simulink model "inverse_kinematics"  (R2021b)
settings: Solver=ode1  StartTime=0.0  StopTime=inf  FixedStep=0.01  RelTol=1e-3
undefined symbols (not defined in the file): Levenberg, Marquardt, W, X, Y, Z
libraries: robotlib x6, simulink x2, robotcorelib x1, robotmaniplib x1
settings Model: Creator=alessandrini  LastModifiedBy=alessandrini
settings SolverCC: AlgebraicLoopSolver=TrustRegion
settings OptimizationCC: EnhancedBackFolding=on  PassReuseOutputArgsThreshold=0  MaxStackSize=64  OptimizeBlockOrder=speed  DifferentSizesBufferReuse=on  OptimizationCustomize=off
settings DebuggingCC: ParameterTunabilityLossMsg=error  SFMachineParentedDataDiag=warning
settings HardwareCC: ProdBitPerPointer=32  ProdBitPerSizeT=32  ProdBitPerPtrDiffT=32  ProdLargestAtomicFloat=None  ProdIntDivRoundTo=Undefined  ProdEndianess=Unspecified  ProdWordSize=32  ProdHWDeviceType=Generic->Unspecified (assume 32-bit Generic)  UseEmbeddedCoderFeatures=off
settings RTWCC: Description=Embedded Coder  SystemTargetFile=ert.tlc  HardwareBoard=Robot Operating System (ROS)  TLCOptions="-aInlineSetEventsForThisBaseRateFcn=TLC_FALSE -aSuppressMultiTaskScheduler=TLC_FALSE  -aRateBasedStepFcn=0"  TemplateMakefile=ert_default_tmf  Toolchain=Catkin  TargetLang=C++
settings CodeAppCC: ForceParamTrailComments=on  OperatorAnnotations=on
settings ERTTargetCC: ERTCustomFileBanners=off  SupportContinuousTime=on  SupportNonInlinedSFcns=on  RemoveResetFunc=off  ModelStepFunctionPrototypeControlCompliant=off

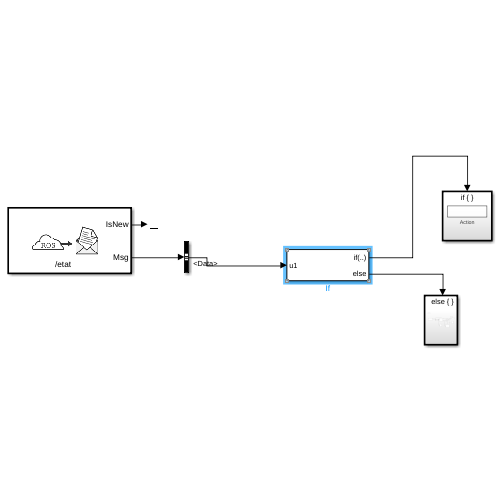
[thumbnail: Simulink's stored preview of the top-level diagram]
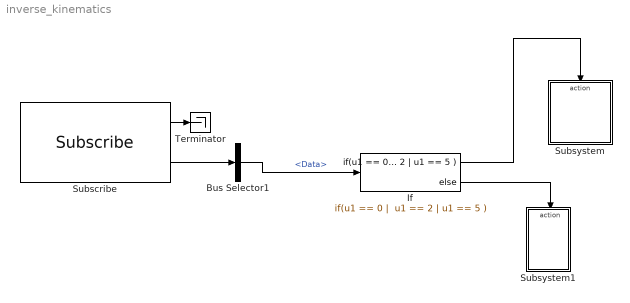
== system inverse_kinematics ==
  Bus Selector1 : BusSelector  OutputSignals=Data
  If : If  IfExpression="u1 == 0 |  u1 == 2 | u1 == 5"
  Subscribe : robotlib/Subscribe  topicSource=Specify your own  topic=/etat  messageType=std_msgs/Int16  SampleTime=-1  legacyBusStruct=off  messageQueueLength=1
  Subsystem : Subsystem
  Subsystem1 : Subsystem
  Terminator : Terminator
  wires:
  Subscribe/2 -> Bus Selector1/1
  Subscribe/1 -> Terminator/1
  Bus Selector1/1 -> If/1  "<Data>"
  If/1 -> Subsystem/Action
  If/2 -> Subsystem1/Action

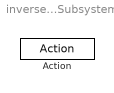
== system inverse_kinematics/Subsystem ==
  Action : ActionPort  InitializeStates=reset  ActionPortLabel="if(u1 == 0 |  u1 == 2 | u1 == 5 )"

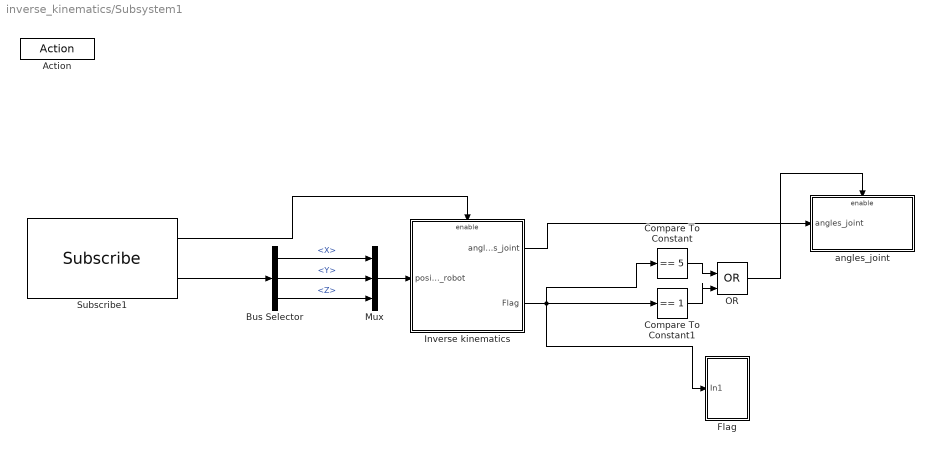
== system inverse_kinematics/Subsystem1 ==
  Action : ActionPort  InitializeStates=reset  ActionPortLabel=else
  Bus Selector : BusSelector  OutputSignals=X,Y,Z
  Compare To Constant : simulink/Logic and Bit Operations/Compare To Constant  relop===  const=5  OutDataTypeStr=boolean
  Compare To Constant1 : simulink/Logic and Bit Operations/Compare To Constant  relop===  const=1  OutDataTypeStr=boolean
  Flag : Subsystem
  Inverse kinematics : Subsystem
  Mux : Mux  Inputs=3
  OR : Logic  Operator=OR  IconShape=distinctive  AllPortsSameDT=off  OutDataTypeStr=boolean
  Subscribe1 : robotlib/Subscribe  topicSource=Specify your own  topic=/position_robot  messageType=geometry_msgs/Point  SampleTime=-1  legacyBusStruct=off  messageQueueLength=10
  angles_joint : Subsystem
  wires:
  Subscribe1/1 -> Inverse kinematics/Enable
  Mux/1 -> Inverse kinematics/1(position_robot)
  Bus Selector/2 -> Mux/2  "<Y>"
  Bus Selector/3 -> Mux/3  "<Z>"
  Inverse kinematics/1(angles_joint) -> angles_joint/1(angles_joint)
  Bus Selector/1 -> Mux/1  "<X>"
  Subscribe1/2 -> Bus Selector/1
  Compare To Constant/1 -> OR/1
  Inverse kinematics/2(Flag) -> Compare To Constant/1, Compare To Constant1/1, Flag/1(In1)
  Compare To Constant1/1 -> OR/2
  OR/1 -> angles_joint/Enable

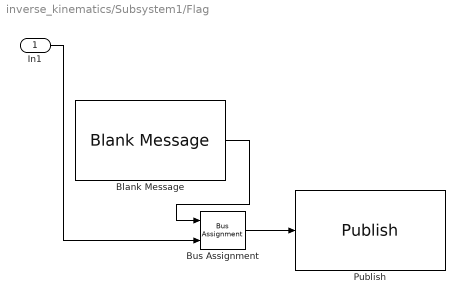
== system inverse_kinematics/Subsystem1/Flag ==
  In1 : Inport
  Blank Message : robotlib/Blank Message  messageClass=Message  entityType=std_msgs/UInt16  messageType=std_msgs/UInt16  SampleTime=-1  legacyBusStruct=off
  Bus Assignment : BusAssignment  AssignedSignals=Data
  Publish : robotlib/Publish  topicSource=Specify your own  topic=/flag  messageType=std_msgs/UInt16  legacyBusStruct=off  messageQueueLength=1
  wires:
  Bus Assignment/1 -> Publish/1
  In1/1 -> Bus Assignment/2
  Blank Message/1 -> Bus Assignment/1

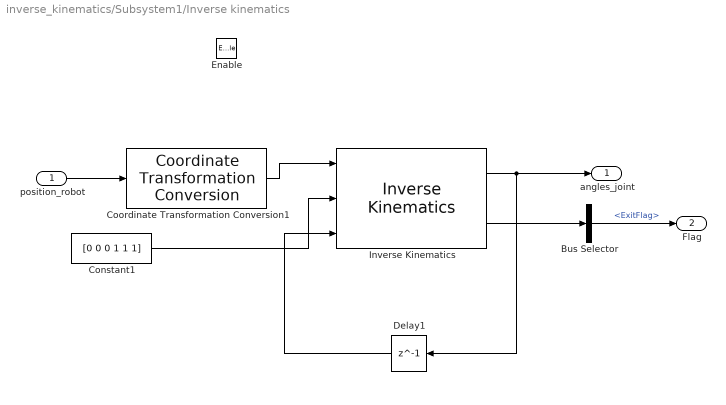
== system inverse_kinematics/Subsystem1/Inverse kinematics ==
  position_robot : Inport
  Enable : EnablePort
  Bus Selector : BusSelector  OutputSignals=ExitFlag
  Constant1 : Constant  Value=[0 0 0 1 1 1]  VectorParams1D=off
  Coordinate Transformation Conversion1 : robotcorelib/Coordinate Transformation Conversion  InputRepresentation=Translation Vector  InputEulerSequence=ZYX  ShowTrVecInputPort=on  OutputRepresentation=Homogeneous Transformation  OutputEulerSequence=ZYX  ShowTrVecOutputPort=on  SimulateUsing=Interpreted execution
  Delay1 : Delay  DelayLength=1  InitialCondition=([19 43 0 -30]*pi/180)'
  Inverse Kinematics : robotmaniplib/Inverse Kinematics  RigidBodyTree=robot  EndEffector=Body5  ShowInfo=on  SolverName=Levenberg-Marquardt  EnforceJointLimits=on  MaxIterations=1500  MaxTime=10  GradientTolerance=1e-7  SolutionTolerance=1e-6  StepTolerance=1e-14  ErrorChangeTolerance=1e-12  UseErrorDamping=on  DampingBias=0.0025  SimulateUsing=Interpreted execution
  angles_joint : Outport
  Flag : Outport  Port=2
  wires:
  Inverse Kinematics/1 -> Delay1/1, angles_joint/1
  Inverse Kinematics/2 -> Bus Selector/1
  position_robot/1 -> Coordinate Transformation Conversion1/1
  Constant1/1 -> Inverse Kinematics/2
  Coordinate Transformation Conversion1/1 -> Inverse Kinematics/1
  Delay1/1 -> Inverse Kinematics/3
  Bus Selector/1 -> Flag/1  "<ExitFlag>"

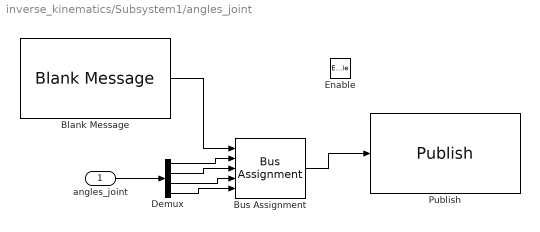
== system inverse_kinematics/Subsystem1/angles_joint ==
  angles_joint : Inport
  Enable : EnablePort
  Blank Message : robotlib/Blank Message  messageClass=Message  entityType=geometry_msgs/Quaternion  messageType=geometry_msgs/Quaternion  SampleTime=-1  legacyBusStruct=off
  Bus Assignment : BusAssignment  AssignedSignals=X,Y,Z,W
  Demux : Demux
  Publish : robotlib/Publish  topicSource=Specify your own  topic=/angles_joint_limit  messageType=geometry_msgs/Quaternion  legacyBusStruct=off  messageQueueLength=1
  wires:
  Bus Assignment/1 -> Publish/1
  Blank Message/1 -> Bus Assignment/1
  Demux/4 -> Bus Assignment/5
  Demux/3 -> Bus Assignment/4
  Demux/2 -> Bus Assignment/3
  Demux/1 -> Bus Assignment/2
  angles_joint/1 -> Demux/1
